simulink model "RIP_simulink"  (R2021a)
settings: Solver=FixedStepAuto  StartTime=0.0  StopTime=100  FixedStep=T  RelTol=1e-3
values from neighbouring files (symbols this model uses):
  Bp = 0.001    [PID_GA.m]    (also in thong_so_dieu_khien_RIP.m; thong_so_dieu_khien_RIP1.m)
  Br = 0.1    [PID_GA.m]    (also in thong_so_dieu_khien_RIP.m)
  Jm = 2.52e-5    (= 2.52e-05)    [PID_GA.m]    (also in thong_so_dieu_khien_RIP.m; thong_so_dieu_khien_RIP1.m)
  Kb = 0.07    [PID_GA.m]    (also in thong_so_dieu_khien_RIP.m; thong_so_dieu_khien_RIP1.m)
  kd1 = par(bestchrom,3)-100    [PID_GA.m]    (also in test_PID.m = 0.35; thong_so_dieu_khien_RIP1.m = 0)
  kd2 = par(bestchrom,6)-100    [PID_GA.m]    (also in test_PID.m = 3.9; thong_so_dieu_khien_RIP1.m = 0)
  ki1 = par(bestchrom,2)-100    [PID_GA.m]    (also in thong_so_dieu_khien_RIP1.m = 0)
  ki2 = par(bestchrom,5)-100    [PID_GA.m]    (also in thong_so_dieu_khien_RIP1.m = 0)
  kp1 = par(bestchrom,1)-100    [PID_GA.m]    (also in test_PID.m = 0.88; thong_so_dieu_khien_RIP1.m = 50)
  kp2 = par(bestchrom,4)-100    [PID_GA.m]    (also in test_PID.m = 46; thong_so_dieu_khien_RIP1.m = 7)
  Kt = 0.07    [PID_GA.m]    (also in thong_so_dieu_khien_RIP.m; thong_so_dieu_khien_RIP1.m)
  Lp = 0.15    [PID_GA.m]    (also in thong_so_dieu_khien_RIP.m; thong_so_dieu_khien_RIP1.m)
  Lr = 0.25    [PID_GA.m]    (also in thong_so_dieu_khien_RIP.m; thong_so_dieu_khien_RIP1.m)
  mp = 0.05388    [PID_GA.m]    (also in thong_so_dieu_khien_RIP.m; thong_so_dieu_khien_RIP1.m)
  mr = 0.2    [PID_GA.m]    (also in thong_so_dieu_khien_RIP.m; thong_so_dieu_khien_RIP1.m)
  Rm = 1.7    [PID_GA.m]    (also in thong_so_dieu_khien_RIP.m; thong_so_dieu_khien_RIP1.m)
  T = 0.01    [PID_GA.m]    (also in TestDongLucHoc.m = 1/2*( m_a*va2 + m_p*vp2 + I_a*dth1^2 + I_p*dth2^2 ); thong_so_dieu_khien_RIP.m; thong_so_dieu_khien_RIP1.m)
  x1_init = 0.1    [PID_GA.m]    (also in thong_so_dieu_khien_RIP.m; thong_so_dieu_khien_RIP1.m = 0.314159265359)
  x2_init = 0    [PID_GA.m]    (also in thong_so_dieu_khien_RIP.m = -0.1; thong_so_dieu_khien_RIP1.m = 0.157079632679)
  x3_init = -0.1    [PID_GA.m]    (also in thong_so_dieu_khien_RIP.m = 0; thong_so_dieu_khien_RIP1.m = 0.01)
  x4_init = 0    [PID_GA.m]    (also in thong_so_dieu_khien_RIP.m; thong_so_dieu_khien_RIP1.m = 0.1)
libraries: simulink x2
settings Model: Creator=OS  LastModifiedBy=Lenovo
settings SolverCC: AlgebraicLoopSolver=TrustRegion
settings DebuggingCC: SFMachineParentedDataDiag=warning

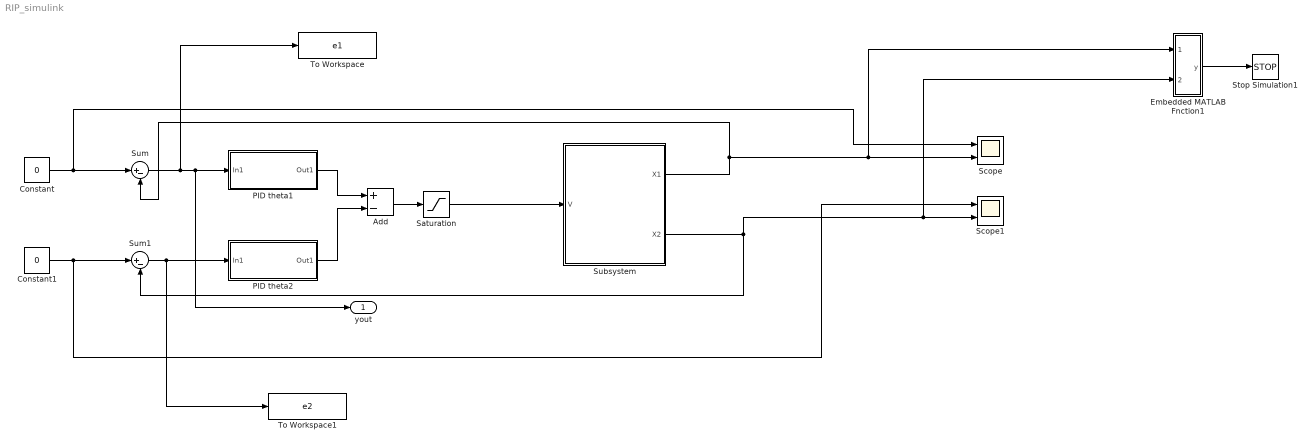
== system RIP_simulink ==
  Add : Sum  Inputs=+-
  Constant : Constant  Value=0
  Constant1 : Constant  Value=0
  Embedded MATLAB Fnction1 : MATLAB Function  TreatAsAtomicUnit=on
  PID theta1 : Subsystem  mask{kp1=kp1, ki1=ki1, kd1=kd1}
  PID theta2 : Subsystem  mask{kp2=kp2, ki2=ki2, kd2=kd2}
  Saturation : Saturate  UpperLimit=24  LowerLimit=-24
  Scope : Scope  NumInputPorts=2
  Scope1 : Scope  NumInputPorts=2
  Stop Simulation1 : Stop
  Subsystem : Subsystem
  Sum : Sum  Inputs=|+-
  Sum1 : Sum  Inputs=|+-
  To Workspace : ToWorkspace  VariableName=e1  SampleTime=0.01
  To Workspace1 : ToWorkspace  VariableName=e2  SampleTime=0.01
  yout : Outport
  wires:
  Sum/1 -> To Workspace/1, yout/1, PID theta1/1(In1)
  Constant/1 -> Scope/1, Sum/1
  PID theta2/1(Out1) -> Add/2
  PID theta1/1(Out1) -> Add/1
  Add/1 -> Saturation/1
  Sum1/1 -> To Workspace1/1, PID theta2/1(In1)
  Constant1/1 -> Scope1/1, Sum1/1
  Embedded MATLAB Fnction1/1(y) -> Stop Simulation1/1
  Saturation/1 -> Subsystem/1(V)
  Subsystem/1(X1) -> Sum/2, Embedded MATLAB Fnction1/1(e1), Scope/2
  Subsystem/2(X2) -> Sum1/2, Embedded MATLAB Fnction1/2(e2), Scope1/2

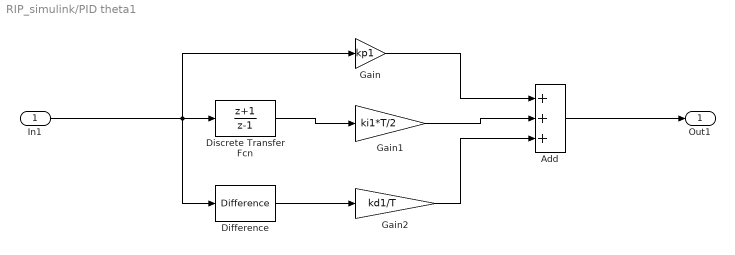
== system RIP_simulink/PID theta1 ==
  In1 : Inport
  Add : Sum  Inputs=+++
  Difference : simulink/Discrete/Difference  ICPrevInput=0.0  OutMin=[]  OutMax=[]  OutDataType=fixdt(1, 16)  OutScaling=2^-10  DoSatur=off
  Discrete Transfer Fcn : DiscreteTransferFcn  Numerator=[1 1]  Denominator=[1 -1]  SampleTime=T
  Gain : Gain  Gain=kp1
  Gain1 : Gain  Gain=ki1*T/2
  Gain2 : Gain  Gain=kd1/T
  Out1 : Outport
  wires:
  Discrete Transfer Fcn/1 -> Gain1/1
  Gain1/1 -> Add/2
  Add/1 -> Out1/1
  Gain/1 -> Add/1
  Gain2/1 -> Add/3
  In1/1 -> Difference/1, Discrete Transfer Fcn/1, Gain/1
  Difference/1 -> Gain2/1

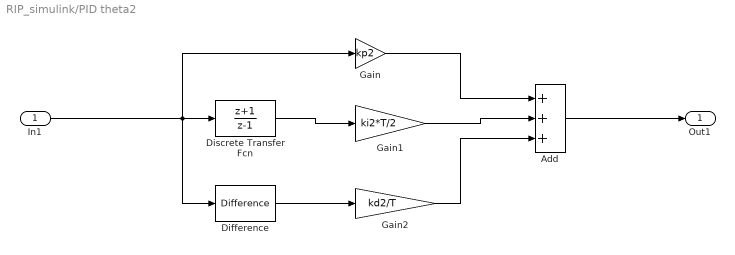
== system RIP_simulink/PID theta2 ==
  In1 : Inport
  Add : Sum  Inputs=+++
  Difference : simulink/Discrete/Difference  ICPrevInput=0.0  OutMin=[]  OutMax=[]  OutDataType=fixdt(1, 16)  OutScaling=2^-10  DoSatur=off
  Discrete Transfer Fcn : DiscreteTransferFcn  Numerator=[1 1]  Denominator=[1 -1]  SampleTime=T
  Gain : Gain  Gain=kp2
  Gain1 : Gain  Gain=ki2*T/2
  Gain2 : Gain  Gain=kd2/T
  Out1 : Outport
  wires:
  Difference/1 -> Gain2/1
  Discrete Transfer Fcn/1 -> Gain1/1
  Gain/1 -> Add/1
  Gain1/1 -> Add/2
  Gain2/1 -> Add/3
  Add/1 -> Out1/1
  In1/1 -> Difference/1, Discrete Transfer Fcn/1, Gain/1

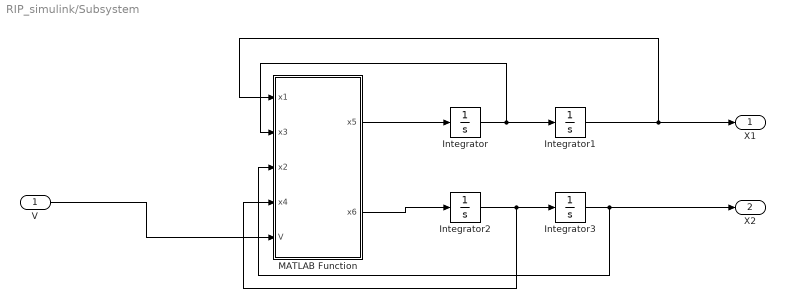
== system RIP_simulink/Subsystem ==
  V : Inport
  Integrator : Integrator  InitialCondition=x3_init
  Integrator1 : Integrator  InitialCondition=x1_init
  Integrator2 : Integrator  InitialCondition=x4_init
  Integrator3 : Integrator  InitialCondition=x2_init
  MATLAB Function : MATLAB Function  TreatAsAtomicUnit=on  mask{Kt=Kt, Kb=Kb, mr=mr, mp=mp, Lp=Lp, Lr=Lr, Br=Br, Bp=Bp, Rm=Rm, Jm=Jm, g=9.81}
  X1 : Outport
  X2 : Outport  Port=2
  wires:
  Integrator1/1 -> MATLAB Function/1(x1), X1/1
  Integrator/1 -> MATLAB Function/2(x3), Integrator1/1
  MATLAB Function/2(x6) -> Integrator2/1
  MATLAB Function/1(x5) -> Integrator/1
  V/1 -> MATLAB Function/5(V)
  Integrator3/1 -> X2/1, MATLAB Function/3(x2)
  Integrator2/1 -> MATLAB Function/4(x4), Integrator3/1

== matlab function RIP_simulink/Embedded MATLAB Fnction1 ==
  data: e1 input; y output; e2 input
function y = fcn(e1,e2)
if (abs(e1)>(3))||(abs(e2)>(3))
    y=1;
else
    y=0;
end

== matlab function RIP_simulink/Subsystem/MATLAB Function ==
  data: x1 input; x3 input; x5 output; x2 input; x4 input; V input; x6 output
function [x5,x6] = fcn(x1,x3,x2,x4,V)
% Thông số của hệ thống 
Kt = 0.07;  % Hằng số momen-xoắn của động cơ 
Kb = 0.07;  % Hằng số điện áp cảm ứng
mr = 0.2;  % Khối lượng của arm 
mp = 0.05388;  % Khối lượng của pendulum 
Lp = 0.15;  % Chiều dài của pendulum 
Lr = 0.25;  % Chiều dài của arm 
Br = 0.1;  % Hệ số cản của arm 
Bp = 0.001;  % Hệ số cản của pendulum
Rm = 1.7;  % Điện trở của động cơ 
Jm = 2.52e-5;  % Hằng số momen quán tính của động cơ 
g = 9.81 ;

x5 =-(6*Br*Lp*Rm*x3 - 6*Kt*Lp*V + 6*Kb*Kt*Lp*x3 + 4*Bp*Lr*Rm*x4*cos(x2) + 3*Lp^3*Rm*mp*x3*x4*sin(2*x2) + 6*Lp^2*Lr*Rm*mp*x4^2*sin(x2) - 2*Lp^2*Lr*Rm*mp*x3^2*sin(2*x2)*cos(x2) - 4*Lp*Lr*Rm*g*mp*cos(x2)*sin(x2))/(Lp*Rm*(6*Jm + 6*Lr^2*mp + 9*Lr^2*mr - 4*Lr^2*mp*cos(x2)^2 + 6*Lp^2*mp*sin(x2)^2));
x6 =(4*Lp^3*Rm*g*mp^2*sin(x2)^3 - 4*Bp*Lr^2*Rm*mp*x4 - 6*Bp*Lr^2*Rm*mr*x4 - 4*Bp*Jm*Rm*x4 + 4*Jm*Lp*Rm*g*mp*sin(x2) + 2*Jm*Lp^2*Rm*mp*x3^2*sin(2*x2) + 2*Lp^4*Rm*mp^2*x3^2*sin(2*x2)*sin(x2)^2 + 4*Lp*Lr^2*Rm*g*mp^2*sin(x2) - 4*Bp*Lp^2*Rm*mp*x4*sin(x2)^2 + 4*Kt*Lp*Lr*V*mp*cos(x2) + 2*Lp^2*Lr^2*Rm*mp^2*x3^2*sin(2*x2) + 3*Lp^2*Lr^2*Rm*mp*mr*x3^2*sin(2*x2) - 4*Br*Lp*Lr*Rm*mp*x3*cos(x2) - 4*Kb*Kt*Lp*Lr*mp*x3*cos(x2) - 4*Lp^2*Lr^2*Rm*mp^2*x4^2*cos(x2)*sin(x2) + 6*Lp*Lr^2*Rm*g*mp*mr*sin(x2) - 2*Lp^3*Lr*Rm*mp^2*x3*x4*sin(2*x2)*cos(x2))/(Lp^2*Rm*mp*(6*Jm + 6*Lr^2*mp + 9*Lr^2*mr - 4*Lr^2*mp*cos(x2)^2 + 6*Lp^2*mp*sin(x2)^2));
end
